simulink model "cs_project"  (R2020a)
settings: Solver=VariableStepAuto  StartTime=0.0  StopTime=50.0  RelTol=1e-3
values from neighbouring files (symbols this model uses):
  A = [-3 0;0 1]    [Untitled.m]    (also in project_code.m = [3 2 3; 3 2 4; 1 1 3])
  B = [0.4 ; 0.3]    [Untitled.m]    (also in project_code.m = [4; 0; 3])
  C = [1 0.4]    [Untitled.m]    (also in project_code.m = [1 1 0.5])
  D = [0]    [Untitled.m]    (also in project_code.m)
  K = place(A,B,controller_eigenvalues)    [Untitled.m]    (also in project_code.m)
  L = place(A',C',observer_eigenvalues)'    [Untitled.m]    (also in project_code.m)
libraries: simulink x2
settings Model: Creator=FAWAD KHAN  LastModifiedBy=FAWAD KHAN

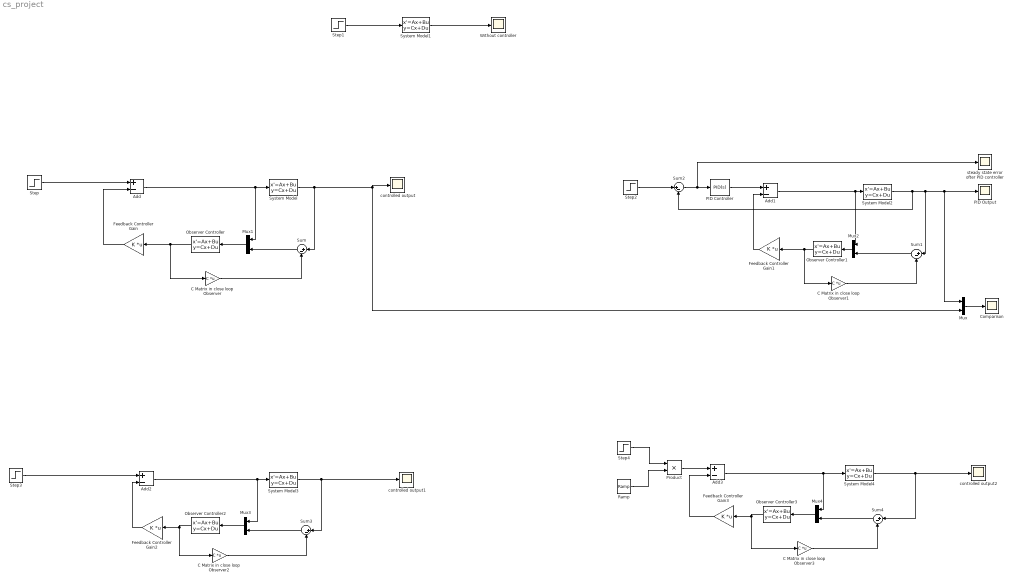
== system cs_project ==
  Add{,1..3} (4 alike) : Sum  Inputs=+-
  C Matrix in close loop Observer{,1..3} (4 alike) : Gain  Gain=C  Multiplication=Matrix(K*u)
  Comparison : Scope
  Feedback Controller Gain{,1..3} (4 alike) : Gain  Gain=K  Multiplication=Matrix(K*u)
  Mux{,1..4} (5 alike) : Mux  Inputs=2
  Observer Controller{,1..3} (4 alike) : StateSpace  A=A  B=[B L]  C=[1 0 0 ;0 1 0;0 0 1 ]  D=[0 0;0 0;0 0]  InitialCondition=0
  PID Controller : simulink/Continuous/PID Controller  Controller=PID  Form=Parallel  TimeDomain=Continuous-time  UseExternalTs=off  SampleTime=-1  IntegratorMethod=Forward Euler  FilterMethod=Forward Euler  ControllerParametersSource=internal  P=0  I=-9.70327032125413  D=0  UseFilter=on  N=100  TunerSelectOption=Transfer Function Based (PID Tuner App)  InitialConditionSource=internal  InitialConditionForIntegrator=0  InitialConditionForFilter=0  DifferentiatorICPrevScaledInput=0  ExternalReset=none  TrackingMode=off  Kt=1  LimitOutput=off  UpperSaturationLimit=inf  LowerSaturationLimit=-inf  LinearizeAsGain=on  AntiWindupMode=none  Kb=1  POutMin=[]  POutMax=[]  IOutMin=[]  IOutMax=[]  DOutMin=[]  DOutMax=[]  NOutMin=[]  NOutMax=[]  SumOutMin=[]  SumOutMax=[]  SaturationOutMin=[]  SaturationOutMax=[]  PParamMin=[]  PParamMax=[]  IParamMin=[]  IParamMax=[]  DParamMin=[]  DParamMax=[]  NParamMin=[]  NParamMax=[]  KbParamMin=[]  KbParamMax=[]  KtParamMin=[]  KtParamMax=[]  KbOutMin=[]  KbOutMax=[]  KtOutMin=[]  KtOutMax=[]  IntegratorOutMin=[]  IntegratorOutMax=[]  FilterOutMin=[]  FilterOutMax=[]  SumI1OutMin=[]  SumI1OutMax=[]  SumI2OutMin=[]  SumI2OutMax=[]  SumI3OutMin=[]  SumI3OutMax=[]  SumI4OutMin=[]  SumI4OutMax=[]  SumDOutMin=[]  SumDOutMax=[]  DifferentiatorOutMin=[]  DifferentiatorOutMax=[]  FilterDiffOutCoefMin=[]  FilterDiffOutCoefMax=[]  ReciprocalOutMin=[]  ReciprocalOutMax=[]  SumDenOutMin=[]  SumDenOutMax=[]  SumNumOutMin=[]  SumNumOutMax=[]  DivideOutMin=[]  DivideOutMax=[]  UdiffTsProdOutMin=[]  UdiffTsProdOutMax=[]  NTsProdOutMin=[]  NTsProdOutMax=[]  UintegralTsProdOutMin=[]  UintegralTsProdOutMax=[]  UngainTsProdOutMin=[]  UngainTsProdOutMax=[]  IntegratorContinuousStateAttributes=''  IntegratorStateMustResolveToSignalObject=off  IntegratorRTWStateStorageClass=Auto  FilterContinuousStateAttributes=''  FilterStateMustResolveToSignalObject=off  FilterRTWStateStorageClass=Auto  ParallelPVariant=InternalParameters  IdealPVariant=Disabled  IVariant=InternalParameters  DVariant=InternalParameters  IntegratorVariant=Continuous  SatVariant=Disabled  AWVariant=Passthrough  PCopyVariant=Disabled  TRVariant=Disabled  FdbkBlocksVariant=Forward  IdealPFdbkVariant=Disabled  SatFdbkVariant=Disabled  DerivativeFilterVariant=ContFilter  NVariant=InternalParameters  NCopyVariant=Disabled  FilterICVariant=InternalICsFilter  IntegratorICVariant=InternalICs  ExternalResetVariant=Disabled  TRSumVariant=Passthrough  SumFdbkVariant=Disabled  SumVariant=Sum_PID  TsampFilterVariant=InternalTs  TsampNgainVariant=Passthrough  TsampIntegralVariant=Passthrough
  PID Output : Scope
  Product : Product
  Ramp : simulink/Sources/Ramp  slope=1  start=0  InitialOutput=0
  Step{,1..2,4} (4 alike) : Step  SampleTime=0
  Step3 : Step  After=2  SampleTime=0
  Sum{,1..4} (5 alike) : Sum  Inputs=|+-
  System Model{,1..4} (5 alike) : StateSpace  A=A  B=B  C=C  D=D  InitialCondition=0
  Without controller : Scope
  controlled output : Scope
  controlled output1 : Scope
  controlled output2 : Scope
  steady state error ofter PID controller : Scope
  wires:
  Step1/1 -> System Model1/1
  System Model1/1 -> Without controller/1
  Mux1/1 -> Observer Controller/1
  Add/1 -> Mux1/1, System Model/1
  Sum/1 -> Mux1/2
  C Matrix in close loop Observer/1 -> Sum/2
  Feedback Controller Gain/1 -> Add/2
  Observer Controller/1 -> C Matrix in close loop Observer/1, Feedback Controller Gain/1
  Observer Controller1/1 -> C Matrix in close loop Observer1/1, Feedback Controller Gain1/1
  PID Controller/1 -> Add1/1
  Feedback Controller Gain1/1 -> Add1/2
  Sum1/1 -> Mux2/2
  C Matrix in close loop Observer1/1 -> Sum1/2
  Add1/1 -> Mux2/1, System Model2/1
  Mux2/1 -> Observer Controller1/1
  Mux/1 -> Comparison/1
  Step2/1 -> Sum2/1
  Sum2/1 -> steady state error ofter PID controller/1, PID Controller/1
  System Model2/1 -> Sum1/1, Mux/1, PID Output/1, Sum2/2
  System Model3/1 -> Sum3/1, controlled output1/1
  C Matrix in close loop Observer2/1 -> Sum3/2
  Mux3/1 -> Observer Controller2/1
  Sum3/1 -> Mux3/2
  Add2/1 -> Mux3/1, System Model3/1
  Feedback Controller Gain2/1 -> Add2/2
  Observer Controller2/1 -> C Matrix in close loop Observer2/1, Feedback Controller Gain2/1
  Add3/1 -> System Model4/1, Mux4/1
  Step4/1 -> Product/1
  C Matrix in close loop Observer3/1 -> Sum4/2
  Observer Controller3/1 -> C Matrix in close loop Observer3/1, Feedback Controller Gain3/1
  Mux4/1 -> Observer Controller3/1
  Sum4/1 -> Mux4/2
  Ramp/1 -> Product/2
  Product/1 -> Add3/1
  Feedback Controller Gain3/1 -> Add3/2
  System Model4/1 -> Sum4/1, controlled output2/1
  Step3/1 -> Add2/1
  Step/1 -> Add/1
  System Model/1 -> Sum/1, Mux/2, controlled output/1
